simulink model "平行接近"  (R2024a)
settings: Solver=ode4  StartTime=0.0  StopTime=inf  FixedStep=0.01  RelTol=1e-3
settings Model: Creator=wenjun  LastModifiedBy=wenjun

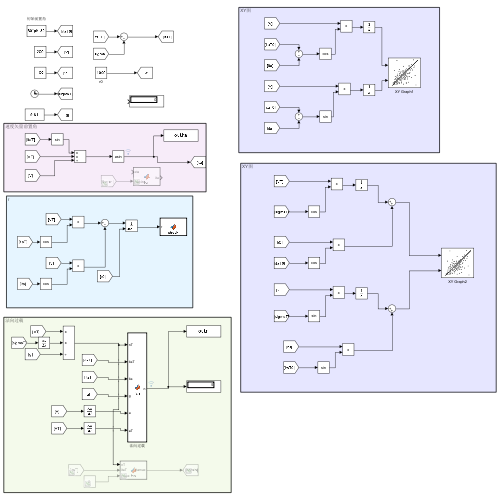
[thumbnail: Simulink's stored preview of the top-level diagram]
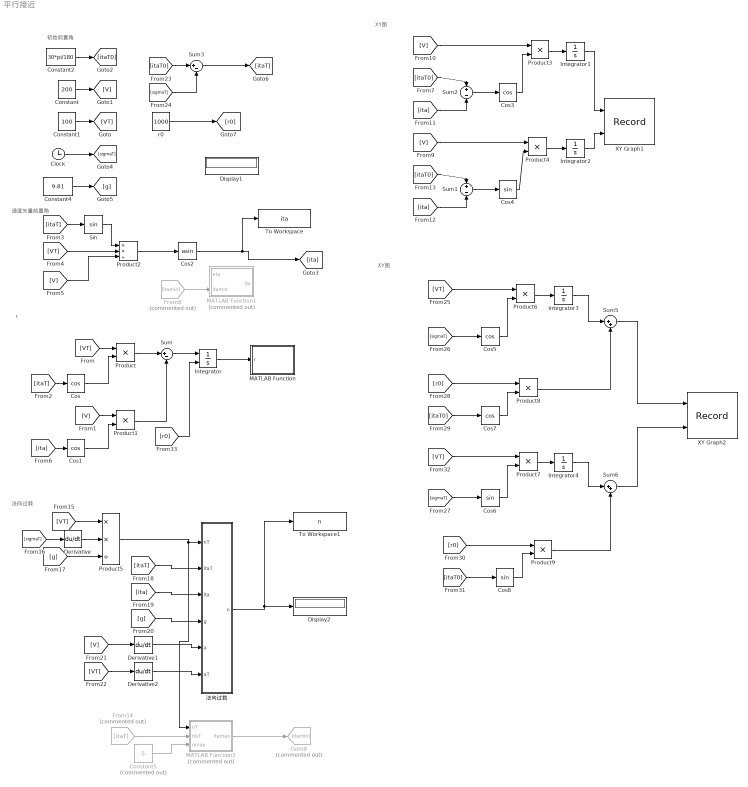
== system 平行接近 ==
  note: 速度矢量前置角
  note: 法向过载
  note: XY图
  note: r
  note: 初始前置角
  note: XY图
  Clock : Clock
  Constant : Constant  Value=200
  Constant1 : Constant  Value=100
  Constant2 : Constant  Value=30*pi/180
  Constant4 : Constant  Value=9.81
  Constant5 : Constant  Commented=on  Value=5
  Cos{,1,3,5,7} (5 alike) : Trigonometry  Operator=cos
  Cos2 : Trigonometry  Operator=asin
  Cos4 : Trigonometry
  Cos6 : Trigonometry
  Cos8 : Trigonometry
  Derivative : Derivative
  Derivative1 : Derivative
  Derivative2 : Derivative
  Display1 : Display
  Display2 : Display
  From14 : From  Commented=on  GotoTag=itaT
  From8 : From  Commented=on  GotoTag=itamin
  Goto8 : Goto  Commented=on  GotoTag=itamin
  Integrator : Integrator  InitialConditionSource=external  InitialCondition=1000
  Integrator{1..4} (4 alike) : Integrator
  MATLAB Function : MATLAB Function  TreatAsAtomicUnit=on
  MATLAB Function1 : MATLAB Function  Commented=on  TreatAsAtomicUnit=on
  MATLAB Function2 : MATLAB Function  Commented=on  TreatAsAtomicUnit=on
  Product{,1,3..4,6..9} (8 alike) : Product
  Product2 : Product  Inputs=**/
  Product5 : Product  Inputs=**/
  Sin : Trigonometry
  Sum : Sum  Inputs=|+-
  Sum1 : Sum  Inputs=+-
  Sum2 : Sum  Inputs=+-
  Sum3 : Sum  Inputs=|+-
  Sum5 : Sum  Inputs=|++
  Sum6 : Sum  Inputs=|++
  To Workspace : ToWorkspace  VariableName=ita  SaveFormat=Timeseries  SampleTime=-1
  To Workspace1 : ToWorkspace  VariableName=n  SaveFormat=Timeseries  SampleTime=-1
  XY Graph1 : Record  VariableName=missileout  RecordToWorkspace=on  FileSettingsInternal="{\"entries\":[{\"content\":{\"excelSettings\":{\"content\":{},\"type\":\"Streamout.ExcelSettings\"}},\"type\":\"Streamout.FileSettingStorage\",\"uuid\":\"\"}],\"packageUris\":[\"http:\\/\\/schema.mathworks.com\\/mf0\\/streamout_blocks\\/R2020a\"],\"version\":\"1.0\"}"  Layout=[1 1]  SignalsInternal="{\"entries\":[{\"content\":{\"signals\":[{\"content\":{\"blockPath\":[],\"dimensions\":[1],\"domain\":\"\",\"lineColor\":\"#64d413\",\"lineWidth\":2,\"plots\":[ 1 ],\"port\":1,\"sid\":[\"\"],\"signalID\":1,\"signalName\":\"Integrator1\"},\"type\":\"RecordBlkView.Signal\",\"uuid\":\"\"},{\"content\":{\"blockPath\":[],\"dimensions\":[1],\"domain\":\"\",\"lineColor\":\"#ff13a6\",\"lineWidth\":2,\"plots\":[ 1 ],\"port\":2,\"sid\":[\"\"],\"signalID\":2,\"signalName\":\"Integrator2\"},\"type\":\"RecordBlkView.Signal\",\"uuid\":\"\"}]},\"type\":\"RecordBlkView.InputSignals\",\"uuid\":\"\"}],\"packageUris\":[\"http:\\/\\/schema.mathworks.com\\/mf0\\/streamout_blocks\\/R2020a\"],\"version\":\"1.0\"}"  VisualizationBindings="{\"xyplotplugin\":{\"info\":[{\"series\":[{\"bindingParametersList\":[{\"parameter\":\"X-Axis\",\"signalID\":1,\"signalName\":\"Integrator1\"},{\"parameter\":\"Y-Axis\",\"signalID\":2,\"signalName\":\"Integrator2\"}],\"seriesID\":0}],\"subplotID\":1}]}}"  CompatibilityTag=XY
  XY Graph2 : Record  VariableName=targetout  RecordToWorkspace=on  FileSettingsInternal="{\"entries\":[{\"content\":{\"excelSettings\":{\"content\":{},\"type\":\"Streamout.ExcelSettings\"}},\"type\":\"Streamout.FileSettingStorage\",\"uuid\":\"\"}],\"packageUris\":[\"http:\\/\\/schema.mathworks.com\\/mf0\\/streamout_blocks\\/R2020a\"],\"version\":\"1.0\"}"  Layout=[1 1]  SignalsInternal="{\"entries\":[{\"content\":{\"signals\":[{\"content\":{\"blockPath\":[],\"dimensions\":[1],\"domain\":\"\",\"lineColor\":\"#ff6929\",\"lineWidth\":2,\"plots\":[ 1 ],\"port\":1,\"sid\":[\"\"],\"signalID\":1,\"signalName\":\"Sum5\"},\"type\":\"RecordBlkView.Signal\",\"uuid\":\"\"},{\"content\":{\"blockPath\":[],\"dimensions\":[1],\"domain\":\"\",\"lineColor\":\"#b746ff\",\"lineWidth\":2,\"plots\":[ 1 ],\"port\":2,\"sid\":[\"\"],\"signalID\":2,\"signalName\":\"Sum6\"},\"type\":\"RecordBlkView.Signal\",\"uuid\":\"\"}]},\"type\":\"RecordBlkView.InputSignals\",\"uuid\":\"\"}],\"packageUris\":[\"http:\\/\\/schema.mathworks.com\\/mf0\\/streamout_blocks\\/R2020a\"],\"version\":\"1.0\"}"  VisualizationBindings="{\"xyplotplugin\":{\"info\":[{\"series\":[{\"bindingParametersList\":[{\"parameter\":\"X-Axis\",\"signalID\":1,\"signalName\":\"Sum5\"},{\"parameter\":\"Y-Axis\",\"signalID\":2,\"signalName\":\"Sum6\"}],\"seriesID\":0}],\"subplotID\":1}]}}"  CompatibilityTag=XY
  r0 : Constant  Value=1000
  法向过载 : MATLAB Function  TreatAsAtomicUnit=on
  wires:
  Constant/1 -> [V]
  Constant1/1 -> [VT]
  [VT] -> Product/1
  Cos/1 -> Product/2
  Product/1 -> Sum/1
  Sum/1 -> Integrator/1
  [V] -> Product1/1
  Cos1/1 -> Product1/2
  Product1/1 -> Sum/2
  [itaT] -> Cos/1
  [itaT] -> Sin/1
  Sin/1 -> Product2/1
  Product2/1 -> Cos2/1
  [VT] -> Product2/2
  [V] -> Product2/3
  [ita] -> Cos1/1
  Constant2/1 -> [itaT0]
  Clock/1 -> [sigmaT]
  Cos3/1 -> Product3/2
  Sum2/1 -> Cos3/1
  [itaT0] -> Sum2/1
  [V] -> Product3/1
  Cos4/1 -> Product4/2
  [itaT0] -> Sum1/1
  [V] -> Product4/1
  Sum1/1 -> Cos4/1
  [r0] -> Integrator/2
  Integrator/1 -> MATLAB Function/1(r)
  [VT] -> Product5/1
  [sigmaT] -> Derivative/1
  Derivative/1 -> Product5/2
  Constant4/1 -> [g]
  [g] -> Product5/3
  Product5/1 -> MATLAB Function2/1(nT), 法向过载/1(nT)
  [itaT] -> 法向过载/2(itaT)
  [ita] -> 法向过载/3(ita)
  [g] -> 法向过载/4(g)
  [V] -> Derivative1/1
  Derivative1/1 -> 法向过载/5(a)
  Derivative2/1 -> 法向过载/6(aT)
  [VT] -> Derivative2/1
  法向过载/1(n) -> To Workspace1/1, Display2/1
  [itaT0] -> Sum3/1
  [sigmaT] -> Sum3/2
  Sum3/1 -> [itaT]
  [sigmaT] -> Cos6/1
  Cos6/1 -> Product7/2
  [sigmaT] -> Cos5/1
  [VT] -> Product6/1
  [VT] -> Product7/1
  Cos5/1 -> Product6/2
  [ita] -> Sum2/2
  [ita] -> Sum1/2
  Cos7/1 -> Product8/2
  [itaT0] -> Cos7/1
  r0/1 -> [r0]
  [r0] -> Product8/1
  Product8/1 -> Sum5/2
  Sum5/1 -> XY Graph2/1
  [itaT0] -> Cos8/1
  Product9/1 -> Sum6/2
  [r0] -> Product9/1
  Cos8/1 -> Product9/2
  Sum6/1 -> XY Graph2/2
  Product3/1 -> Integrator1/1
  Integrator1/1 -> XY Graph1/1
  Product4/1 -> Integrator2/1
  Integrator2/1 -> XY Graph1/2
  Product6/1 -> Integrator3/1
  Integrator3/1 -> Sum5/1
  Product7/1 -> Integrator4/1
  Integrator4/1 -> Sum6/1
  MATLAB Function2/1(itamax) -> Goto8/1
  From8/1 -> MATLAB Function1/2(itamin)
  From14/1 -> MATLAB Function2/2(itaT)
  Constant5/1 -> MATLAB Function2/3(nmax)
  Cos2/1 -> To Workspace/1, [ita]

== matlab function 平行接近/法向过载 ==
  data: nT input; n output; itaT input; ita input; g input; a input; aT input
function n  = fcn(nT,itaT,ita,g,a,aT)

n = nT*cos(itaT)/cos(ita)+(a*sin(ita)/cos(ita)-aT*sin(itaT)/cos(ita))/g;


end

== matlab function 平行接近/MATLAB Function ==
  data: r input
function check(r)

if r <=0
    error('catch up');
end

== matlab function 平行接近/MATLAB Function1 ==
  data: eta input; ita output; itamin input
function ita = fcn(eta,itamin)
if cos(eta)<=itamin
    ita=eta;
else 
    ita=acos(itamin);

end

== matlab function 平行接近/MATLAB Function2 ==
  data: nT input; itamax output; itaT input; nmax input
function itamax = fcn(nT,itaT,nmax)

itamax=nT*cos(itaT)/nmax;
end
